simulink model "cv_2_sim"  (R2019b)
settings: Solver=FixedStepAuto  StartTime=0.0  StopTime=Tsim  FixedStep=Ts  RelTol=1e-3
values from neighbouring files (symbols this model uses):
  a_0 = 9    [cv_2.m]
  a_1 = 6    [cv_2.m]
  dy_0 = 3    [cv_2.m]
  y_0 = 4    [cv_2.m]
undefined symbols (not defined in the file or in its folder): u_0
settings Model: Creator=Martin Dodek  LastModifiedBy=Martin Dodek

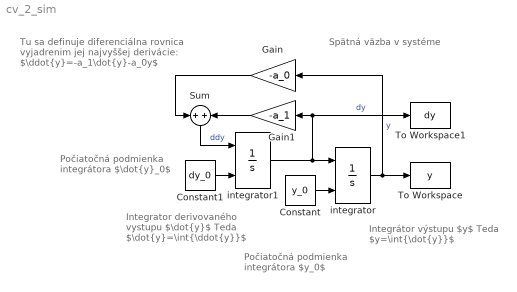
== system cv_2_sim ==
  note: Spätná väzba v systéme
  note: Počiatočná podmienka integrátora
      | $\dot{y}_0$
  note: Tu sa definuje diferenciálna rovnica vyjadrenim jej najvyššej derivácie:
      | $\ddot{y}=-a_1\dot{y}-a_0y$
  note: Počiatočná podmienka integrátora
      | $y_0$
  note: Integrator derivovaného vystupu $\dot{y}$
      | Teda $\dot{y}=\int{\ddot{y}}$
  note: Integrátor výstupu $y$
      | Teda $y=\int{\dot{y}}$
  Constant : Constant  Value=y_0
  Constant1 : Constant  Value=dy_0
  Gain : Gain  Gain=-a_0
  Gain1 : Gain  Gain=-a_1
  Sum : Sum
  To Workspace : ToWorkspace  VariableName=y  SampleTime=-1
  To Workspace1 : ToWorkspace  VariableName=dy  SampleTime=-1
  integrator : Integrator  InitialConditionSource=external  InitialCondition=u_0
  integrator1 : Integrator  InitialConditionSource=external  InitialCondition=u_0
  wires:
  Constant/1 -> integrator/2
  integrator/1 -> To Workspace/1, Gain/1  "y"
  integrator1/1 -> To Workspace1/1, Gain1/1, integrator/1  "dy"
  Constant1/1 -> integrator1/2
  Sum/1 -> integrator1/1  "ddy"
  Gain/1 -> Sum/1
  Gain1/1 -> Sum/2
